simulink library "basic_create_THB"  (Simulink 8.2)
settings: Solver=ode45  StartTime=0.0  StopTime=10.0  RelTol=1e-3
undefined symbols (not defined in the file): dia, fluid, mID, mix, p
libraries: carnot x3
settings Model: Creator=lena.frank  LastModifiedBy=drhf

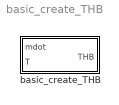
== system basic_create_THB ==
  basic_create_THB : Subsystem  mask(create THV){p=p, fluid=fluid, mix=mix, dia=dia, hgt=0, mID=mID}
      mask prompts: p "pressure [Pa]"; mix "fluid mixture [0..1]"; dia "diameter [m]"; hgt "Geodetic height in m"; mID "Calculation mode"
      mask help:
      | Create a THB with the variable input T and mdot. The other value can be set as constants in the mask.
      | Calculation mode:
      |     1 ..  9999 no pressure drop (dp)
      | 10001 .. 19999 dp caused by flowrate
      | 20001 .. inf   dp by flowrate and static height
      mask init:
      | mix = min(1, max(0, mix));
      | dia = max(dia, 0.001);
      mask Help: web(fullfile(path_carnot('help'),'basic_create_THB.html'),'-helpbrowser')

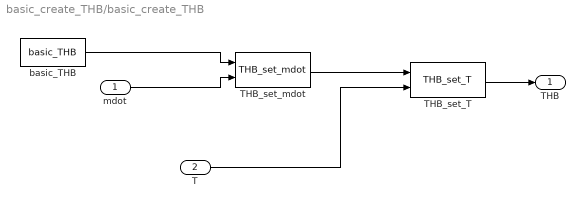
== system basic_create_THB/basic_create_THB ==
  mdot : Inport
  T : Inport  Port=2
  THB_set_T : carnot/Source/Simple/THB_set_T
  THB_set_mdot : carnot/Source/Simple/THB_set_mdot
  basic_THB : carnot/Basic/Hydraulics/basic_THB  t=10  mdot=0  p=p  ID=1  fluid=fluid  mix=mix  dia=dia  hgt=hgt
  THB : Outport
  wires:
  basic_THB/1 -> THB_set_mdot/1
  mdot/1 -> THB_set_mdot/2
  THB_set_mdot/1 -> THB_set_T/1
  THB_set_T/1 -> THB/1
  T/1 -> THB_set_T/2
